simulink model "HDLHeaderSeparate"  (R2024a)
settings: Solver=VariableStepAuto  StartTime=0.0  StopTime=stopTime  RelTol=1e-3
undefined symbols (not defined in the file): CONST
libraries: HDL_ieee_8021513 x3, dspsrcs4 x2
settings Model: Creator=cotti  LastModifiedBy=cotti

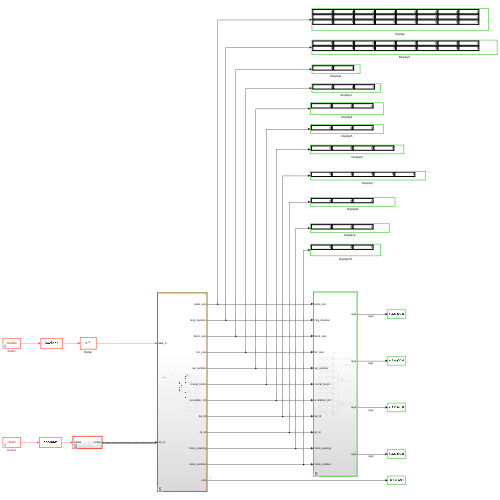
[thumbnail: Simulink's stored preview of the top-level diagram]
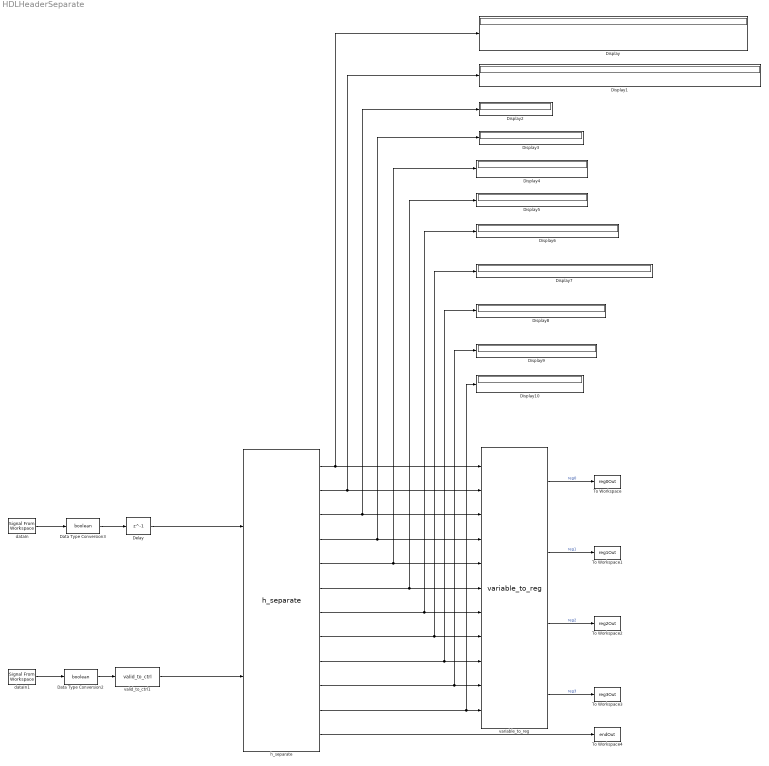
== system HDLHeaderSeparate ==
  Data Type Conversion2 : DataTypeConversion  OutDataTypeStr=boolean  SaturateOnIntegerOverflow=off  RndMeth=Floor
  Data Type Conversion3 : DataTypeConversion  OutDataTypeStr=boolean  SaturateOnIntegerOverflow=off  RndMeth=Floor
  Delay : Delay  DelayLength=1  InitialCondition=0  UseCircularBuffer=on
  Display{,1..10} (11 alike) : Display
  To Workspace : ToWorkspace  VariableName=reg0Out  SampleTime=4/CONST.fPHY
      settings: Save2DSignal=2-D array (concatenate along first dimension)
  To Workspace1 : ToWorkspace  VariableName=reg1Out  SampleTime=4/CONST.fPHY
      settings: Save2DSignal=2-D array (concatenate along first dimension)
  To Workspace2 : ToWorkspace  VariableName=reg2Out  SampleTime=4/CONST.fPHY
      settings: Save2DSignal=2-D array (concatenate along first dimension)
  To Workspace3 : ToWorkspace  VariableName=reg3Out  SampleTime=4/CONST.fPHY
      settings: Save2DSignal=2-D array (concatenate along first dimension)
  To Workspace4 : ToWorkspace  VariableName=endOut  SampleTime=4/CONST.fPHY
      settings: Save2DSignal=2-D array (concatenate along first dimension)
  dataIn : dspsrcs4/Signal From Workspace  X=dataBits  Ts=1/CONST.fs  nsamps=1  OutputAfterFinalValue=Setting to zero  ignoreOrWarnInputAndFrameLengths=off  OutputFrames=off
  dataIn1 : dspsrcs4/Signal From Workspace  X=validIn  Ts=1/CONST.fs  nsamps=1  OutputAfterFinalValue=Setting to zero  ignoreOrWarnInputAndFrameLengths=off  OutputFrames=off
  h_separate : HDL_ieee_8021513/h_separate  SystemSampleTime=-1  VariantActivationTime=update diagram  AllowFlexibleInterface=on  Latency=0  AutoFrameSizeCalculation=off
      settings: SourceProductName=HDL IEEE 8021513
  valid_to_ctrl1 : HDL_ieee_8021513/valid_to_ctrl  SystemSampleTime=-1  VariantActivationTime=update diagram  AllowFlexibleInterface=on  Latency=0  AutoFrameSizeCalculation=off
      settings: SourceProductName=HDL IEEE 8021513
  variable_to_reg : HDL_ieee_8021513/variable_to_reg  SystemSampleTime=-1  VariantActivationTime=update diagram  AllowFlexibleInterface=on  Latency=0  AutoFrameSizeCalculation=off
      settings: SourceProductName=HDL IEEE 8021513
  wires:
  h_separate/11 -> variable_to_reg/11, Display10/1
  h_separate/10 -> variable_to_reg/10, Display9/1
  h_separate/9 -> variable_to_reg/9, Display8/1
  h_separate/8 -> variable_to_reg/8, Display7/1
  h_separate/7 -> variable_to_reg/7, Display6/1
  h_separate/6 -> variable_to_reg/6, Display5/1
  h_separate/5 -> variable_to_reg/5, Display4/1
  h_separate/4 -> variable_to_reg/4, Display3/1
  h_separate/3 -> variable_to_reg/3, Display2/1
  h_separate/2 -> variable_to_reg/2, Display1/1
  h_separate/1 -> variable_to_reg/1, Display/1
  dataIn1/1 -> Data Type Conversion2/1
  valid_to_ctrl1/1 -> h_separate/2
  Data Type Conversion2/1 -> valid_to_ctrl1/1
  dataIn/1 -> Data Type Conversion3/1
  Delay/1 -> h_separate/1
  Data Type Conversion3/1 -> Delay/1
  variable_to_reg/1 -> To Workspace/1  "reg0"
  variable_to_reg/2 -> To Workspace1/1  "reg1"
  variable_to_reg/3 -> To Workspace2/1  "reg2"
  variable_to_reg/4 -> To Workspace3/1  "reg3"
  h_separate/12 -> To Workspace4/1
